simulink model "gm_lab2_fixp"  (R2022a)
settings: Solver=VariableStepAuto  StartTime=0.0  StopTime=10.0  RelTol=1e-3
settings Model: Creator=user  LastModifiedBy=user
settings OptimizationCC: BlockReduction=off  ConditionallyExecuteInputs=off
settings DebuggingCC: InheritedTsInSrcMsg=none

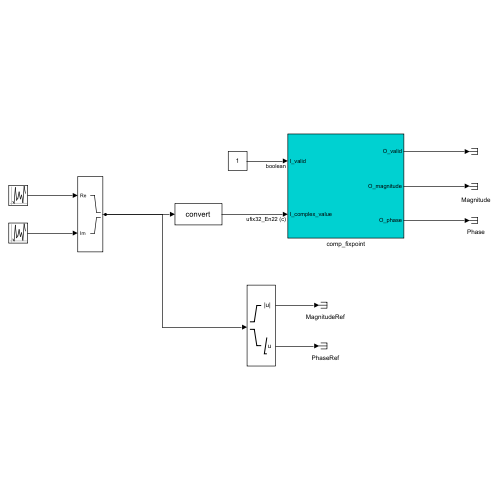
[thumbnail: Simulink's stored preview of the top-level diagram]
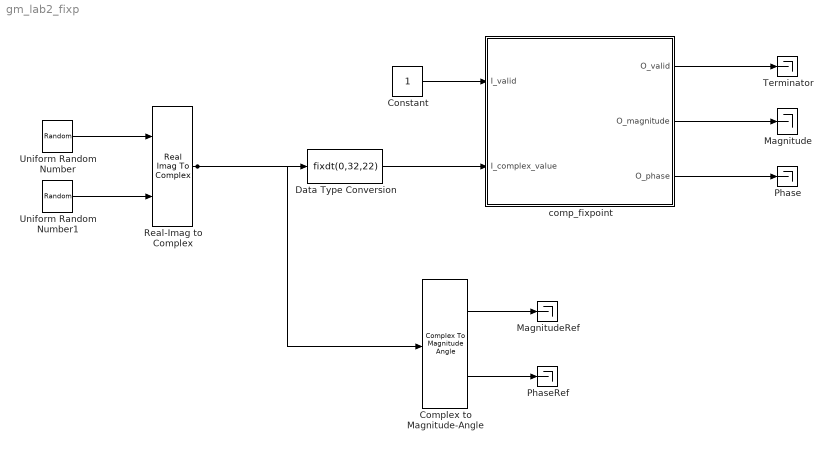
== system gm_lab2_fixp ==
  Complex to Magnitude-Angle : ComplexToMagnitudeAngle
  Constant : Constant  OutDataTypeStr=boolean  SampleTime=1
  Data Type Conversion : DataTypeConversion  OutDataTypeStr=fixdt(0,32,22)  RndMeth=Round
  Magnitude : Terminator
  MagnitudeRef : Terminator
  Phase : Terminator
  PhaseRef : Terminator
  Real-Imag to Complex : RealImagToComplex
  Terminator : Terminator
  Uniform Random Number : UniformRandomNumber  Minimum=0  Maximum=1023.99999976158142089844  Seed=10  SampleTime=1
  Uniform Random Number1 : UniformRandomNumber  Minimum=0  Maximum=1023.99999976158142089844  Seed=11  SampleTime=1
  comp_fixpoint : Subsystem
  wires:
  Complex to Magnitude-Angle/2 -> PhaseRef/1
  Complex to Magnitude-Angle/1 -> MagnitudeRef/1
  comp_fixpoint/2(O_magnitude) -> Magnitude/1
  comp_fixpoint/3(O_phase) -> Phase/1
  Data Type Conversion/1 -> comp_fixpoint/2(I_complex_value)
  comp_fixpoint/1(O_valid) -> Terminator/1
  Constant/1 -> comp_fixpoint/1(I_valid)
  Real-Imag to Complex/1 -> Data Type Conversion/1, Complex to Magnitude-Angle/1
  Uniform Random Number/1 -> Real-Imag to Complex/1
  Uniform Random Number1/1 -> Real-Imag to Complex/2

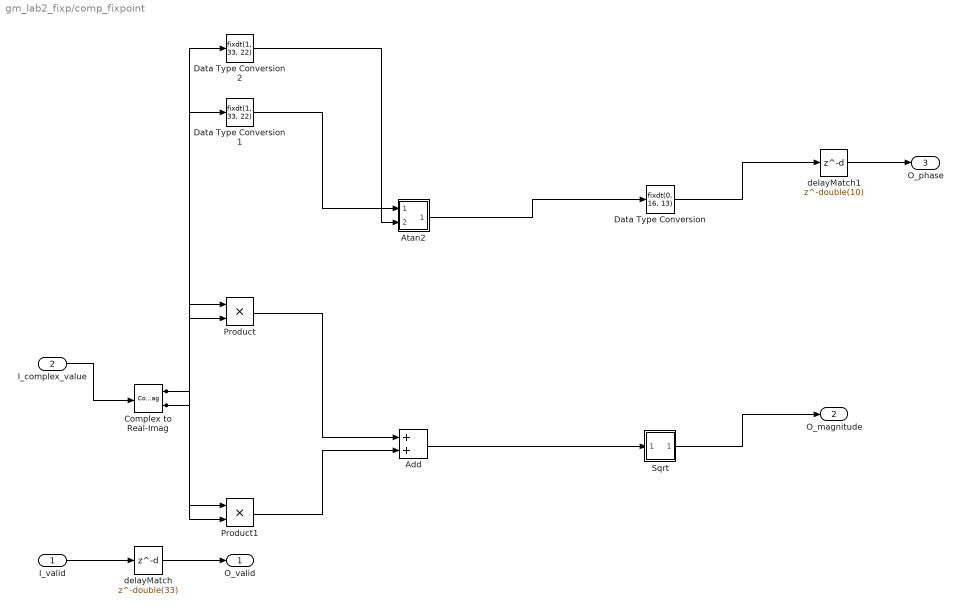
== system gm_lab2_fixp/comp_fixpoint ==
  I_valid : Inport  OutDataTypeStr=boolean  PortDimensions=1  SampleTime=1
  I_complex_value : Inport  Port=2  OutDataTypeStr=fixdt(0, 32, 22)  PortDimensions=1  SampleTime=1
      settings: SignalType=complex
  Add : Sum  AccumDataTypeStr=fixdt(0, 64, 44)  OutDataTypeStr=fixdt(0, 64, 44)  SampleTime=1
  Atan2 : Subsystem
  Complex to Real-Imag : ComplexToRealImag  SampleTime=1
  Data Type Conversion : DataTypeConversion  OutDataTypeStr=fixdt(0, 16, 13)  RndMeth=Round  SampleTime=1  SaturateOnIntegerOverflow=off
  Data Type Conversion1 : DataTypeConversion  OutDataTypeStr=fixdt(1, 33, 22)  SampleTime=1  SaturateOnIntegerOverflow=off  RndMeth=Floor
  Data Type Conversion2 : DataTypeConversion  OutDataTypeStr=fixdt(1, 33, 22)  SampleTime=1  SaturateOnIntegerOverflow=off  RndMeth=Floor
  Product : Product  Inputs=**  OutDataTypeStr=fixdt(0, 64, 44)  SampleTime=1
  Product1 : Product  Inputs=**  OutDataTypeStr=fixdt(0, 64, 44)  SampleTime=1
  Sqrt : Subsystem
  delayMatch : Delay  DelayLength=double(33)  InitialCondition=0  SampleTime=1
  delayMatch1 : Delay  DelayLength=double(10)  InitialCondition=0  SampleTime=1
  O_valid : Outport  SampleTime=1
  O_magnitude : Outport  Port=2  SampleTime=1
  O_phase : Outport  Port=3  SampleTime=1
  wires:
  delayMatch/1 -> O_valid/1
  I_complex_value/1 -> Complex to Real-Imag/1
  Add/1 -> Sqrt/1(In1)
  Atan2/1(Out1) -> Data Type Conversion/1
  Complex to Real-Imag/1 -> Product/2, Product/1, Data Type Conversion2/1
  Complex to Real-Imag/2 -> Product1/2, Product1/1, Data Type Conversion1/1
  delayMatch1/1 -> O_phase/1
  Data Type Conversion1/1 -> Atan2/1(In1)
  Data Type Conversion2/1 -> Atan2/2(In2)
  Product/1 -> Add/1
  Product1/1 -> Add/2
  Sqrt/1(Out1) -> O_magnitude/1
  I_valid/1 -> delayMatch/1
  Data Type Conversion/1 -> delayMatch1/1

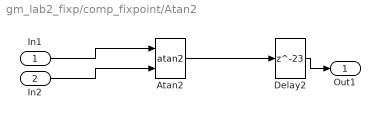
== system gm_lab2_fixp/comp_fixpoint/Atan2 ==
  In1 : Inport
  In2 : Inport  Port=2
  Atan2 : Trigonometry  Operator=atan2  ApproximationMethod=CORDIC  NumberOfIterations=20
  Delay2 : Delay  DelayLength=23
  Out1 : Outport
  wires:
  In1/1 -> Atan2/1
  In2/1 -> Atan2/2
  Atan2/1 -> Delay2/1
  Delay2/1 -> Out1/1

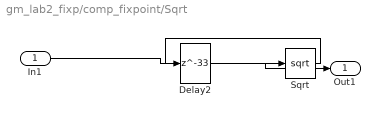
== system gm_lab2_fixp/comp_fixpoint/Sqrt ==
  In1 : Inport
  Delay2 : Delay  DelayLength=33
  Sqrt : Sqrt  OutDataTypeStr=fixdt(0,33,21)
  Out1 : Outport
  wires:
  In1/1 -> Sqrt/1
  Sqrt/1 -> Delay2/1
  Delay2/1 -> Out1/1
